simulink model "SILPILexternoselavededavide"  (R2023b)
settings: Solver=FixedStepDiscrete  StartTime=0.0  StopTime=10.0  FixedStep=Ts  RelTol=1e-3
values from neighbouring files (symbols this model uses):
  sys_discrete_motor = c2d(sys_continuos_motor,0.005,'tustin')    [model_approximation.m]
  Ts = 0.005    [attempt.m]    (also in model_approximation.m; tuning.m)
settings Model: Creator=giova  LastModifiedBy=giova

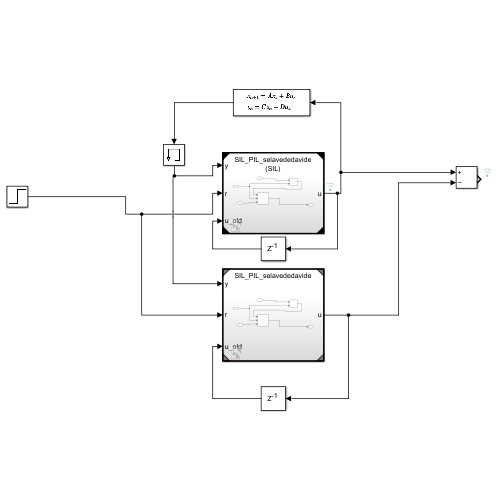
[thumbnail: Simulink's stored preview of the top-level diagram]
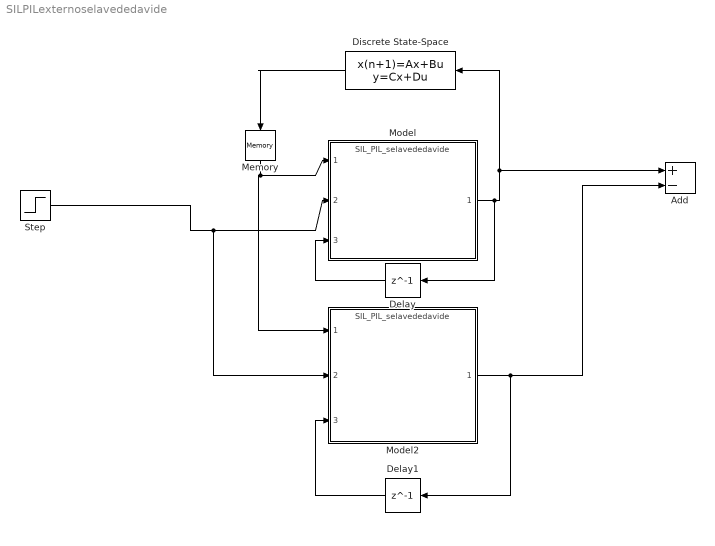
== system SILPILexternoselavededavide ==
  Add : Sum  Inputs=+-
  Delay : Delay  DelayLength=1
  Delay1 : Delay  DelayLength=1
  Discrete State-Space : DiscreteStateSpace  A=sys_discrete_motor.A  B=sys_discrete_motor.B  C=sys_discrete_motor.C  D=sys_discrete_motor.D  InitialCondition=[0 0 0]  SampleTime=Ts
  Memory : Memory
  Model : ModelReference  ModelNameDialog=SIL_PIL_selavededavide.slx  SimulationMode=Software-in-the-loop (SIL)  ModelReferenceVersion=1.6
  Model2 : ModelReference  ModelNameDialog=SIL_PIL_selavededavide.slx  SimulationMode=Normal  ModelReferenceVersion=1.6
  Step : Step  Time=0  After=3.14
  wires:
  Step/1 -> Model2/2, Model/2
  Model/1 -> Delay/1, Discrete State-Space/1, Add/1
  Discrete State-Space/1 -> Memory/1
  Model2/1 -> Delay1/1, Add/2
  Delay/1 -> Model/3
  Delay1/1 -> Model2/3
  Memory/1 -> Model2/1, Model/1
